simulink model "robotarm_A2_breach"  (R2018b)
settings: Solver=FixedStepAuto  StartTime=0.0  StopTime=tspan(end)  RelTol=1e-3  AbsTol=1e-6
undefined symbols (not defined in the file): options
libraries: neural x132, simulink x2
(part 2 of 6)

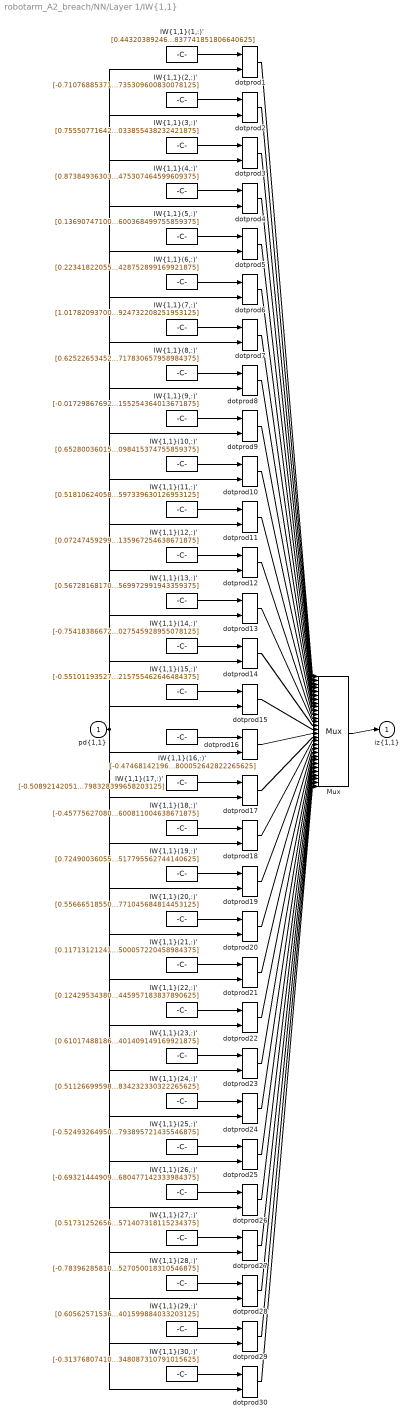
== system robotarm_A2_breach/NN/Layer 1/IW{1,1} ==
  "pd{1,1}" : Inport  PortDimensions=10
      mask Display: e = 0.06;c1 = [120 230 180]/255;c2 = ([120 230 180]+0)/(256+128);c3 = ([120 230 180]+128)/(256+128);patch([0 1 1 0],[0 0 1 1],c1);patch([0 1 1 1-e 1-e 0+e],[0 0 1 1-e 0+e 0+e],c2);patch([0 0 1 1-e 0+e 0+e],[0 1 1 1-e 1-e 0+e],c3);plot([0 1 1 0 0],[0 0 1 1 0]);
  "IW{1,1}(1,:)'" : Constant  Value=[0.44320389246650415682182710952474735677242279052734375;0.51947584556928483312532307536457665264606475830078125;-0.1013749825861565978524225783985457383096218109130859375;-0.465941513924777728217208050409681163728237152099609375;0.67801884953176971837507380769238807260990142822265625;-0.81570216281103657962603392661549150943756103515625;0.80632098302361898678469742662855423986911773681640625;0.01324690942009895851250167453372341697104275226593017578125;-0.64580771410095449969190894989878870546817779541015625;-0.76009607664536960047740876689204014837741851806640625]
      mask Display: e = 0.06;c1 = [120 150 230]/255;c2 = ([120 150 230]+0)/383;c3 = ([120 150 230]+128)/383;patch([0 1 1 0],[0 0 1 1],c1);patch([0 1 1 1-e 1-e 0+e],[0 0 1 1-e 0+e 0+e],c2);patch([0 0 1 1-e 0+e 0+e],[0 1 1 1-e 1-e 0+e],c3);plot([0 1 1 0 0],[0 0 1 1 0]);disp('Weights');
  "IW{1,1}(10,:)'" : Constant  Value=[0.6528003601570897540540272530051879584789276123046875;-0.805642874886827176084125312627293169498443603515625;-0.016554816769301171353045987189034349285066127777099609375;0.76137713758309855105466112945578061044216156005859375;-0.7006051933474084503217227393179200589656829833984375;0.7652873118121277240533117947052232921123504638671875;0.51417600395731877238603146906825713813304901123046875;0.247761309628450943076671819653711281716823577880859375;0.349447996093606771950135225779376924037933349609375;0.8974588918394699188496588249108754098415374755859375]
      mask Display: e = 0.06;c1 = [120 150 230]/255;c2 = ([120 150 230]+0)/383;c3 = ([120 150 230]+128)/383;patch([0 1 1 0],[0 0 1 1],c1);patch([0 1 1 1-e 1-e 0+e],[0 0 1 1-e 0+e 0+e],c2);patch([0 0 1 1-e 0+e 0+e],[0 1 1 1-e 1-e 0+e],c3);plot([0 1 1 0 0],[0 0 1 1 0]);disp('Weights');
  "IW{1,1}(11,:)'" : Constant  Value=[0.51810624058172383143983097397722303867340087890625;0.872191799817235047243002554751001298427581787109375;-0.712884895735269363825636901310645043849945068359375;0.002494892009457406502337395437507439055480062961578369140625;-0.270486052055616099654145045860786922276020050048828125;0.6707615472857841876219708865392021834850311279296875;0.0246310505931925417810735012835721136070787906646728515625;0.77266353199085024971992652353947050869464874267578125;-0.3568298560395135599065952192177064716815948486328125;0.360121164362003032266557056573219597339630126953125]
      mask Display: e = 0.06;c1 = [120 150 230]/255;c2 = ([120 150 230]+0)/383;c3 = ([120 150 230]+128)/383;patch([0 1 1 0],[0 0 1 1],c1);patch([0 1 1 1-e 1-e 0+e],[0 0 1 1-e 0+e 0+e],c2);patch([0 0 1 1-e 0+e 0+e],[0 1 1 1-e 1-e 0+e],c3);plot([0 1 1 0 0],[0 0 1 1 0]);disp('Weights');
  "IW{1,1}(12,:)'" : Constant  Value=[0.07247459299068963189949243997034500353038311004638671875;0.77588832922420791771145331949810497462749481201171875;-0.01498952312966151008410964351469374378211796283721923828125;-0.66950481581926502006041346248821355402469635009765625;-1.0394647414620890035763522973866201937198638916015625;0.41659107015939067508725202060304582118988037109375;-0.56564242470902581505498574188095517456531524658203125;0.772999076426951869933645866694860160350799560546875;-0.15300878050934751950507006768020801246166229248046875;0.46525515641211512285480011996696703135967254638671875]
      mask Display: e = 0.06;c1 = [120 150 230]/255;c2 = ([120 150 230]+0)/383;c3 = ([120 150 230]+128)/383;patch([0 1 1 0],[0 0 1 1],c1);patch([0 1 1 1-e 1-e 0+e],[0 0 1 1-e 0+e 0+e],c2);patch([0 0 1 1-e 0+e 0+e],[0 1 1 1-e 1-e 0+e],c3);plot([0 1 1 0 0],[0 0 1 1 0]);disp('Weights');
  "IW{1,1}(13,:)'" : Constant  Value=[0.56728168170493098454443270384217612445354461669921875;0.277793118270089234300712632830254733562469482421875;-0.5975587782155187266397433631937019526958465576171875;0.06833884407195851828920041270976071245968341827392578125;-0.856917725762365467545578212593682110309600830078125;0.7908637356047483191190394791192375123500823974609375;-0.06487009020830931949053166363228228874504566192626953125;0.2372887359075701863009300041085225529968738555908203125;-0.2256653137890034799273308863121201284229755401611328125;0.8783771195165426259876539916149340569972991943359375]
      mask Display: e = 0.06;c1 = [120 150 230]/255;c2 = ([120 150 230]+0)/383;c3 = ([120 150 230]+128)/383;patch([0 1 1 0],[0 0 1 1],c1);patch([0 1 1 1-e 1-e 0+e],[0 0 1 1-e 0+e 0+e],c2);patch([0 0 1 1-e 0+e 0+e],[0 1 1 1-e 1-e 0+e],c3);plot([0 1 1 0 0],[0 0 1 1 0]);disp('Weights');
  "IW{1,1}(14,:)'" : Constant  Value=[-0.75418386672222437194790245484909974038600921630859375;1.1398123201737184739812391853774897754192352294921875;-0.58445642008161347025207987826433964073657989501953125;0.164696959702814005321869217368657700717449188232421875;-0.73703910480042511554898965187021531164646148681640625;0.471437080031712529848419990230468101799488067626953125;0.59769416587250834282940559205599129199981689453125;0.018010030288912466656103816831091535277664661407470703125;-0.377438339776456188712216999192605726420879364013671875;0.111431025352921431181840716817532666027545928955078125]
      mask Display: e = 0.06;c1 = [120 150 230]/255;c2 = ([120 150 230]+0)/383;c3 = ([120 150 230]+128)/383;patch([0 1 1 0],[0 0 1 1],c1);patch([0 1 1 1-e 1-e 0+e],[0 0 1 1-e 0+e 0+e],c2);patch([0 0 1 1-e 0+e 0+e],[0 1 1 1-e 1-e 0+e],c3);plot([0 1 1 0 0],[0 0 1 1 0]);disp('Weights');
  "IW{1,1}(15,:)'" : Constant  Value=[-0.55101193527417435813475776740233413875102996826171875;0.0671325813779753699517272025332204066216945648193359375;-0.60519616319179825314478193831746466457843780517578125;0.58769100257684769861299400872667320072650909423828125;-0.08797219520669753711761273962110863067209720611572265625;-0.5524094229546279155584898035158403217792510986328125;-0.7448941576311882695193844483583234250545501708984375;0.81814789464563464349566856981255114078521728515625;0.5804459365944396598280263788183219730854034423828125;0.8181125456554683150756090981303714215755462646484375]
      mask Display: e = 0.06;c1 = [120 150 230]/255;c2 = ([120 150 230]+0)/383;c3 = ([120 150 230]+128)/383;patch([0 1 1 0],[0 0 1 1],c1);patch([0 1 1 1-e 1-e 0+e],[0 0 1 1-e 0+e 0+e],c2);patch([0 0 1 1-e 0+e 0+e],[0 1 1 1-e 1-e 0+e],c3);plot([0 1 1 0 0],[0 0 1 1 0]);disp('Weights');
  "IW{1,1}(16,:)'" : Constant  Value=[-0.4746814219666923850837747522746212780475616455078125;0.94193468075639363856765839955187402665615081787109375;-0.81513375864305803730758270830847322940826416015625;-0.5388084969969246795784556525177322328090667724609375;-0.1592610235542184782264740761092980392277240753173828125;-0.0600385525680668108439164143419475294649600982666015625;-0.329608468077444427546396354955504648387432098388671875;0.584753683074171082267866950132884085178375244140625;-0.51700864122426237745600019479752518236637115478515625;-0.78562921103160709979107423350797034800052642822265625]
      mask Display: e = 0.06;c1 = [120 150 230]/255;c2 = ([120 150 230]+0)/383;c3 = ([120 150 230]+128)/383;patch([0 1 1 0],[0 0 1 1],c1);patch([0 1 1 1-e 1-e 0+e],[0 0 1 1-e 0+e 0+e],c2);patch([0 0 1 1-e 0+e 0+e],[0 1 1 1-e 1-e 0+e],c3);plot([0 1 1 0 0],[0 0 1 1 0]);disp('Weights');
  "IW{1,1}(17,:)'" : Constant  Value=[-0.50892142051125277557588333365856669843196868896484375;-0.69555083700712694305678951423033140599727630615234375;0.60851594624274041311906557893962599337100982666015625;-1.0252220281550294966876890612184070050716400146484375;-0.2168840042489936503766756459299358539283275604248046875;0.6757041508143555308407712800544686615467071533203125;0.479959671170491375402633593694190494716167449951171875;-0.792943564626870767142463591881096363067626953125;0.1627362166961741907211802526944666169583797454833984375;0.0198821736009527801070095875957122188992798328399658203125]
      mask Display: e = 0.06;c1 = [120 150 230]/255;c2 = ([120 150 230]+0)/383;c3 = ([120 150 230]+128)/383;patch([0 1 1 0],[0 0 1 1],c1);patch([0 1 1 1-e 1-e 0+e],[0 0 1 1-e 0+e 0+e],c2);patch([0 0 1 1-e 0+e 0+e],[0 1 1 1-e 1-e 0+e],c3);plot([0 1 1 0 0],[0 0 1 1 0]);disp('Weights');
  "IW{1,1}(18,:)'" : Constant  Value=[-0.4577562708069302654934062957181595265865325927734375;1.2676395565921485530935797214624471962451934814453125;0.364524994376268285378728251089341938495635986328125;0.316539673426614542872670199358253739774227142333984375;0.1632538241122458988474619445696589536964893341064453125;0.49761099855925594592775951241492293775081634521484375;-0.748043169166599408725915054674260318279266357421875;0.275886447527427247639053575767320580780506134033203125;-0.27855783778322640298341639208956621587276458740234375;0.46158990380921494089960788187454454600811004638671875]
      mask Display: e = 0.06;c1 = [120 150 230]/255;c2 = ([120 150 230]+0)/383;c3 = ([120 150 230]+128)/383;patch([0 1 1 0],[0 0 1 1],c1);patch([0 1 1 1-e 1-e 0+e],[0 0 1 1-e 0+e 0+e],c2);patch([0 0 1 1-e 0+e 0+e],[0 1 1 1-e 1-e 0+e],c3);plot([0 1 1 0 0],[0 0 1 1 0]);disp('Weights');
  "IW{1,1}(19,:)'" : Constant  Value=[0.724900360550514211155359589611180126667022705078125;-0.74523780018478535946968577263760380446910858154296875;-0.47796223974658491595590703582274727523326873779296875;0.322867547667288146140407434359076432883739471435546875;0.50749193517804369601975622572354041039943695068359375;0.79033776973074820748621505117625929415225982666015625;-0.4530942934193140647636255380348302423954010009765625;-0.499085576358067106728100270629511214792728424072265625;0.139279961878759628302049122794414870440959930419921875;0.2482889911062852450474025545190670527517795562744140625]
      mask Display: e = 0.06;c1 = [120 150 230]/255;c2 = ([120 150 230]+0)/383;c3 = ([120 150 230]+128)/383;patch([0 1 1 0],[0 0 1 1],c1);patch([0 1 1 1-e 1-e 0+e],[0 0 1 1-e 0+e 0+e],c2);patch([0 0 1 1-e 0+e 0+e],[0 1 1 1-e 1-e 0+e],c3);plot([0 1 1 0 0],[0 0 1 1 0]);disp('Weights');
  "IW{1,1}(2,:)'" : Constant  Value=[-0.71076885371394282753243487604777328670024871826171875;-0.7199239242746739986245074760518036782741546630859375;0.60890423360056422641406470575020648539066314697265625;-0.8359265181922317378138131971354596316814422607421875;-0.01236466893263855719442556591047832625918090343475341796875;-0.086936016752006739505276300405967049300670623779296875;-0.83008311124606082298527098828344605863094329833984375;-0.708547490288692127791136954328976571559906005859375;-0.372731541127455046069627542237867601215839385986328125;0.6533615363197065040168354244087822735309600830078125]
      mask Display: e = 0.06;c1 = [120 150 230]/255;c2 = ([120 150 230]+0)/383;c3 = ([120 150 230]+128)/383;patch([0 1 1 0],[0 0 1 1],c1);patch([0 1 1 1-e 1-e 0+e],[0 0 1 1-e 0+e 0+e],c2);patch([0 0 1 1-e 0+e 0+e],[0 1 1 1-e 1-e 0+e],c3);plot([0 1 1 0 0],[0 0 1 1 0]);disp('Weights');
  "IW{1,1}(20,:)'" : Constant  Value=[0.5566651855048128094693993261898867785930633544921875;-0.44166086307228591412155083162360824644565582275390625;0.047687377290480836844466239199391566216945648193359375;-0.58969305305443875386828267437522299587726593017578125;-0.27878213042887522998825033937464468181133270263671875;0.95487524421580893818628510416601784527301788330078125;-0.3976653837847201611310765656526200473308563232421875;0.2471805959416451814458781655048369430005550384521484375;-0.18325039106971008351365526323206722736358642578125;0.5749228586424852682768005252000875771045684814453125]
      mask Display: e = 0.06;c1 = [120 150 230]/255;c2 = ([120 150 230]+0)/383;c3 = ([120 150 230]+128)/383;patch([0 1 1 0],[0 0 1 1],c1);patch([0 1 1 1-e 1-e 0+e],[0 0 1 1-e 0+e 0+e],c2);patch([0 0 1 1-e 0+e 0+e],[0 1 1 1-e 1-e 0+e],c3);plot([0 1 1 0 0],[0 0 1 1 0]);disp('Weights');
  "IW{1,1}(21,:)'" : Constant  Value=[0.11713121241022854401858666051339241676032543182373046875;-0.161379468950165361196269486754317767918109893798828125;-0.7571548590667889211403007720946334302425384521484375;-0.5838206531095664342245754596660844981670379638671875;-0.239675887371985696372433949363767169415950775146484375;-0.4271977908733119999595828630845062434673309326171875;-0.5864204481509058819455049160751514136791229248046875;0.832557507211043823502905070199631154537200927734375;-0.43356891709465716910898436253773979842662811279296875;-0.6054667698450602042470336527912877500057220458984375]
      mask Display: e = 0.06;c1 = [120 150 230]/255;c2 = ([120 150 230]+0)/383;c3 = ([120 150 230]+128)/383;patch([0 1 1 0],[0 0 1 1],c1);patch([0 1 1 1-e 1-e 0+e],[0 0 1 1-e 0+e 0+e],c2);patch([0 0 1 1-e 0+e 0+e],[0 1 1 1-e 1-e 0+e],c3);plot([0 1 1 0 0],[0 0 1 1 0]);disp('Weights');
  "IW{1,1}(22,:)'" : Constant  Value=[0.1242953438074253791345569197801523841917514801025390625;0.8801330808879919143095094113959930837154388427734375;-0.63780439820036083364840351350721903145313262939453125;-0.33948603439440550033623367198742926120758056640625;0.4331515967100065811479225885705091059207916259765625;0.78263969117551901444329587320680730044841766357421875;0.361190678789260755099377320220810361206531524658203125;-0.89372467515034514917715569026768207550048828125;-0.6160858098907056046300567686557769775390625;-0.1207696284431253597180244696573936380445957183837890625]
      mask Display: e = 0.06;c1 = [120 150 230]/255;c2 = ([120 150 230]+0)/383;c3 = ([120 150 230]+128)/383;patch([0 1 1 0],[0 0 1 1],c1);patch([0 1 1 1-e 1-e 0+e],[0 0 1 1-e 0+e 0+e],c2);patch([0 0 1 1-e 0+e 0+e],[0 1 1 1-e 1-e 0+e],c3);plot([0 1 1 0 0],[0 0 1 1 0]);disp('Weights');
  "IW{1,1}(23,:)'" : Constant  Value=[0.61017488186100854452575958930538035929203033447265625;0.1706451267918588643457411535564460791647434234619140625;-0.458039832655668111005553555514779873192310333251953125;-0.65247583865402258851418082485906779766082763671875;0.5436317432158996876268020059796981513500213623046875;-0.57938981805185096884969198072212748229503631591796875;0.6548718804419044747788802851573564112186431884765625;0.1616631179037730514647108748249593190848827362060546875;-0.727430760154359479230379292857833206653594970703125;0.541767729955985100076532035018317401409149169921875]
      mask Display: e = 0.06;c1 = [120 150 230]/255;c2 = ([120 150 230]+0)/383;c3 = ([120 150 230]+128)/383;patch([0 1 1 0],[0 0 1 1],c1);patch([0 1 1 1-e 1-e 0+e],[0 0 1 1-e 0+e 0+e],c2);patch([0 0 1 1-e 0+e 0+e],[0 1 1 1-e 1-e 0+e],c3);plot([0 1 1 0 0],[0 0 1 1 0]);disp('Weights');
  "IW{1,1}(24,:)'" : Constant  Value=[0.51126699598210845199020013751578517258167266845703125;0.2474125636719124166074124104852671734988689422607421875;0.7825633408629191212213527251151390373706817626953125;0.401031003354632542556856833471101708710193634033203125;0.40237460000039659835380234653712250292301177978515625;0.428379990475945049421824251112411729991436004638671875;0.78279557710397240644084604355157352983951568603515625;-0.79848599732739600209896480009774677455425262451171875;-0.164755224531509092411596384408767335116863250732421875;-0.54600511891358627369896794334636069834232330322265625]
      mask Display: e = 0.06;c1 = [120 150 230]/255;c2 = ([120 150 230]+0)/383;c3 = ([120 150 230]+128)/383;patch([0 1 1 0],[0 0 1 1],c1);patch([0 1 1 1-e 1-e 0+e],[0 0 1 1-e 0+e 0+e],c2);patch([0 0 1 1-e 0+e 0+e],[0 1 1 1-e 1-e 0+e],c3);plot([0 1 1 0 0],[0 0 1 1 0]);disp('Weights');
  "IW{1,1}(25,:)'" : Constant  Value=[-0.524932649501538950431722696521319448947906494140625;-0.648777122723714239072023701737634837627410888671875;0.0307647862348335542070909554013269371353089809417724609375;0.6454191306393770588556435541249811649322509765625;-0.5017327542510103821626898934482596814632415771484375;0.99523431649100546625419383417465724050998687744140625;-0.75566215465000008411067256020032800734043121337890625;-0.070746109627535691544153451104648411273956298828125;-0.01490998250299602201351945041096769273281097412109375;-0.52465858272687693197866565242293290793895721435546875]
      mask Display: e = 0.06;c1 = [120 150 230]/255;c2 = ([120 150 230]+0)/383;c3 = ([120 150 230]+128)/383;patch([0 1 1 0],[0 0 1 1],c1);patch([0 1 1 1-e 1-e 0+e],[0 0 1 1-e 0+e 0+e],c2);patch([0 0 1 1-e 0+e 0+e],[0 1 1 1-e 1-e 0+e],c3);plot([0 1 1 0 0],[0 0 1 1 0]);disp('Weights');
  "IW{1,1}(26,:)'" : Constant  Value=[-0.69321444909777196752287409253767691552639007568359375;0.310984724690046399064868865025346167385578155517578125;-0.69058813895924486825350641083787195384502410888671875;-0.70125747804459270806631820960319600999355316162109375;0.27626987322017981796307140029966831207275390625;-0.284795830435694174997962591078248806297779083251953125;0.038821887770207667844868382189815747551620006561279296875;-0.71972748404353625861773480210104025900363922119140625;-0.39656616262824850860368997018667869269847869873046875;-0.73129209094150071646112110101967118680477142333984375]
      mask Display: e = 0.06;c1 = [120 150 230]/255;c2 = ([120 150 230]+0)/383;c3 = ([120 150 230]+128)/383;patch([0 1 1 0],[0 0 1 1],c1);patch([0 1 1 1-e 1-e 0+e],[0 0 1 1-e 0+e 0+e],c2);patch([0 0 1 1-e 0+e 0+e],[0 1 1 1-e 1-e 0+e],c3);plot([0 1 1 0 0],[0 0 1 1 0]);disp('Weights');
  "IW{1,1}(27,:)'" : Constant  Value=[0.5173125265682563256319781430647708475589752197265625;-0.049397491354776119909519849215939757414162158966064453125;-0.81740761486488278109163729823194444179534912109375;-0.08412318439210035581066193799415486864745616912841796875;0.1553109267276908955768277564857271499931812286376953125;0.17722402391180158698347213430679403245449066162109375;-0.90548653814202573197889023504103533923625946044921875;0.41262963643356564968911470714374445378780364990234375;1.087835541343836087690988279064185917377471923828125;0.56545162151599848154859273563488386571407318115234375]
      mask Display: e = 0.06;c1 = [120 150 230]/255;c2 = ([120 150 230]+0)/383;c3 = ([120 150 230]+128)/383;patch([0 1 1 0],[0 0 1 1],c1);patch([0 1 1 1-e 1-e 0+e],[0 0 1 1-e 0+e 0+e],c2);patch([0 0 1 1-e 0+e 0+e],[0 1 1 1-e 1-e 0+e],c3);plot([0 1 1 0 0],[0 0 1 1 0]);disp('Weights');
  "IW{1,1}(28,:)'" : Constant  Value=[-0.78396285810341759248132120774243958294391632080078125;-0.00910046633940105216542537647228527930565178394317626953125;-0.66004759121113687481141596435918472707271575927734375;-0.78043938724562778030957588271121494472026824951171875;-0.2491602188595275768623338308316306211054325103759765625;0.68534921788892899652267942656180821359157562255859375;-0.0069191367098792866396905765213887207210063934326171875;-0.84621331274527544774599618904176168143749237060546875;0.5373132351323077759985835655243135988712310791015625;0.62345550018999773556060972623527050018310546875]
      mask Display: e = 0.06;c1 = [120 150 230]/255;c2 = ([120 150 230]+0)/383;c3 = ([120 150 230]+128)/383;patch([0 1 1 0],[0 0 1 1],c1);patch([0 1 1 1-e 1-e 0+e],[0 0 1 1-e 0+e 0+e],c2);patch([0 0 1 1-e 0+e 0+e],[0 1 1 1-e 1-e 0+e],c3);plot([0 1 1 0 0],[0 0 1 1 0]);disp('Weights');
  "IW{1,1}(29,:)'" : Constant  Value=[0.60562571536392340032506353963981382548809051513671875;-0.532825242205438254217142457491718232631683349609375;0.82195499843903763181884869482018984854221343994140625;-0.1673989818227205883527375362973543815314769744873046875;0.68771892273064205713950514109455980360507965087890625;-0.09491219601184143483951771713691414333879947662353515625;-0.48907899718634617602930347857181914150714874267578125;0.34930477962741812714142497497959993779659271240234375;-0.497850007887704337772305507314740680158138275146484375;1.07647261589812348603345526498742401599884033203125]
      mask Display: e = 0.06;c1 = [120 150 230]/255;c2 = ([120 150 230]+0)/383;c3 = ([120 150 230]+128)/383;patch([0 1 1 0],[0 0 1 1],c1);patch([0 1 1 1-e 1-e 0+e],[0 0 1 1-e 0+e 0+e],c2);patch([0 0 1 1-e 0+e 0+e],[0 1 1 1-e 1-e 0+e],c3);plot([0 1 1 0 0],[0 0 1 1 0]);disp('Weights');
  "IW{1,1}(3,:)'" : Constant  Value=[0.75550771642954728246621698417584411799907684326171875;0.4651970624553471989059971747337840497493743896484375;0.316389969701839135485244014489580877125263214111328125;0.95234081392340019789344296441413462162017822265625;-0.54512424096975220511041015925002284348011016845703125;-0.1199486488292370311992129927602945826947689056396484375;-0.489955622693164671854759717462002299726009368896484375;-0.25132352667878044005789206494227983057498931884765625;0.1268370320189154132339837133258697576820850372314453125;-0.744428647658245790097453209455125033855438232421875]
      mask Display: e = 0.06;c1 = [120 150 230]/255;c2 = ([120 150 230]+0)/383;c3 = ([120 150 230]+128)/383;patch([0 1 1 0],[0 0 1 1],c1);patch([0 1 1 1-e 1-e 0+e],[0 0 1 1-e 0+e 0+e],c2);patch([0 0 1 1-e 0+e 0+e],[0 1 1 1-e 1-e 0+e],c3);plot([0 1 1 0 0],[0 0 1 1 0]);disp('Weights');
  "IW{1,1}(30,:)'" : Constant  Value=[-0.313768074103874361480137622493202798068523406982421875;-0.617033842266395904374576275586150586605072021484375;0.410502019716686927797155703956377692520618438720703125;0.81012929193932325944160766084678471088409423828125;-0.043151646587668519849945170108185266144573688507080078125;0.0210179663767442910515814702421266702003777027130126953125;-0.424715750473314390678325480621424503624439239501953125;0.88620338133446885375832380304927937686443328857421875;-0.7949468812020141772478609709651209414005279541015625;0.93967254890675688816514821155578829348087310791015625]
      mask Display: e = 0.06;c1 = [120 150 230]/255;c2 = ([120 150 230]+0)/383;c3 = ([120 150 230]+128)/383;patch([0 1 1 0],[0 0 1 1],c1);patch([0 1 1 1-e 1-e 0+e],[0 0 1 1-e 0+e 0+e],c2);patch([0 0 1 1-e 0+e 0+e],[0 1 1 1-e 1-e 0+e],c3);plot([0 1 1 0 0],[0 0 1 1 0]);disp('Weights');
  "IW{1,1}(4,:)'" : Constant  Value=[0.87384936303111848676650197376147843897342681884765625;-0.2287493200660979109084536275986465625464916229248046875;-0.241602336087604452341537353277090005576610565185546875;-0.1587639918776705127978488008011481724679470062255859375;-0.95146944816727463400951592120691202580928802490234375;-0.60279055737714148932582247653044760227203369140625;0.6273114429944215419965303226490505039691925048828125;0.57828806947814526129292289624572731554508209228515625;0.34936344574905942028664185272646136581897735595703125;-0.023795202179214401672080470007131225429475307464599609375]
      mask Display: e = 0.06;c1 = [120 150 230]/255;c2 = ([120 150 230]+0)/383;c3 = ([120 150 230]+128)/383;patch([0 1 1 0],[0 0 1 1],c1);patch([0 1 1 1-e 1-e 0+e],[0 0 1 1-e 0+e 0+e],c2);patch([0 0 1 1-e 0+e 0+e],[0 1 1 1-e 1-e 0+e],c3);plot([0 1 1 0 0],[0 0 1 1 0]);disp('Weights');
  "IW{1,1}(5,:)'" : Constant  Value=[0.1369074710004203609958750575970043428242206573486328125;-0.1139511764867985055271759620154625736176967620849609375;1.0525915567382597703982582970638759434223175048828125;-0.298822917521910202953705493200686760246753692626953125;-0.97249453951210573787733437711722217500209808349609375;0.79674479353023475169948142138309776782989501953125;-0.1330203219585482099507345310485106892883777618408203125;-0.6436253507153135711149616327020339667797088623046875;0.266075168516050009070994519788655452430248260498046875;0.02548060304491460426046245402176282368600368499755859375]
      mask Display: e = 0.06;c1 = [120 150 230]/255;c2 = ([120 150 230]+0)/383;c3 = ([120 150 230]+128)/383;patch([0 1 1 0],[0 0 1 1],c1);patch([0 1 1 1-e 1-e 0+e],[0 0 1 1-e 0+e 0+e],c2);patch([0 0 1 1-e 0+e 0+e],[0 1 1 1-e 1-e 0+e],c3);plot([0 1 1 0 0],[0 0 1 1 0]);disp('Weights');
  "IW{1,1}(6,:)'" : Constant  Value=[0.2234182205573691515354539660620503127574920654296875;-0.86690746220813375000346923116012476384639739990234375;0.94444867744370719631064048371626995503902435302734375;1.074067905807680300966922004590742290019989013671875;0.2481737568000013383073820705249090678989887237548828125;-0.261006977650531102330688781876233406364917755126953125;-0.380288866215888032851211164597771130502223968505859375;-0.25353732613580215460302724750363267958164215087890625;0.638937860708570948276019407785497605800628662109375;0.1333282944150208926270551046400214545428752899169921875]
      mask Display: e = 0.06;c1 = [120 150 230]/255;c2 = ([120 150 230]+0)/383;c3 = ([120 150 230]+128)/383;patch([0 1 1 0],[0 0 1 1],c1);patch([0 1 1 1-e 1-e 0+e],[0 0 1 1-e 0+e 0+e],c2);patch([0 0 1 1-e 0+e 0+e],[0 1 1 1-e 1-e 0+e],c3);plot([0 1 1 0 0],[0 0 1 1 0]);disp('Weights');
  "IW{1,1}(7,:)'" : Constant  Value=[1.017820937001784553643801700673066079616546630859375;0.40855130381393911509491090328083373606204986572265625;0.397315672322906709990064655357855372130870819091796875;0.01521358336158879810684485534011400886811316013336181640625;0.07800441716808721726028608145497855730354785919189453125;-0.1554513220874771117774315598580869846045970916748046875;0.5621451195729696426184318625018931925296783447265625;0.7946680824603458148658319259993731975555419921875;0.53650469033950487496298364931135438382625579833984375;-0.51599999329390844327036802496877498924732208251953125]
      mask Display: e = 0.06;c1 = [120 150 230]/255;c2 = ([120 150 230]+0)/383;c3 = ([120 150 230]+128)/383;patch([0 1 1 0],[0 0 1 1],c1);patch([0 1 1 1-e 1-e 0+e],[0 0 1 1-e 0+e 0+e],c2);patch([0 0 1 1-e 0+e 0+e],[0 1 1 1-e 1-e 0+e],c3);plot([0 1 1 0 0],[0 0 1 1 0]);disp('Weights');
  "IW{1,1}(8,:)'" : Constant  Value=[0.62522653452871035373306085602962411940097808837890625;-0.62499448228666754090454560355283319950103759765625;-0.6579888802018782900660198720288462936878204345703125;0.417744195494852477157365910898079164326190948486328125;-0.717550952346133197323752028751187026500701904296875;0.4652313896980599938757450217963196337223052978515625;-0.7028735615850560947137637413106858730316162109375;0.269824973790782574045721275979303754866123199462890625;-0.80052495489638175740765291266143321990966796875;0.2878933218308306063448753775446675717830657958984375]
      mask Display: e = 0.06;c1 = [120 150 230]/255;c2 = ([120 150 230]+0)/383;c3 = ([120 150 230]+128)/383;patch([0 1 1 0],[0 0 1 1],c1);patch([0 1 1 1-e 1-e 0+e],[0 0 1 1-e 0+e 0+e],c2);patch([0 0 1 1-e 0+e 0+e],[0 1 1 1-e 1-e 0+e],c3);plot([0 1 1 0 0],[0 0 1 1 0]);disp('Weights');
  "IW{1,1}(9,:)'" : Constant  Value=[-0.0172986769296754640257152146887165145017206668853759765625;-0.5329186140946335914492237861850298941135406494140625;0.61939908834851842289737078317557461559772491455078125;-0.329992727773426308690574160209507681429386138916015625;-1.0193204469705381409738720321911387145519256591796875;0.81164190044688344638501575900590978562831878662109375;-0.11180129901829237437649311459608725272119045257568359375;0.36683924979239213026716015519923530519008636474609375;-0.6534477435602068506881323628476820886135101318359375;-0.05659662109145240094232320871014962904155254364013671875]
      mask Display: e = 0.06;c1 = [120 150 230]/255;c2 = ([120 150 230]+0)/383;c3 = ([120 150 230]+128)/383;patch([0 1 1 0],[0 0 1 1],c1);patch([0 1 1 1-e 1-e 0+e],[0 0 1 1-e 0+e 0+e],c2);patch([0 0 1 1-e 0+e 0+e],[0 1 1 1-e 1-e 0+e],c3);plot([0 1 1 0 0],[0 0 1 1 0]);disp('Weights');
  Mux : Mux  Inputs=30
      mask Display: e = 0.06;c1 = [120 150 230]/255;c2 = ([120 150 230]+0)/383;c3 = ([120 150 230]+128)/383;patch([0 1 1 0],[0 0 1 1],c1);patch([0 1 1 1-e 1-e 0+e],[0 0 1 1-e 0+e 0+e],c2);patch([0 0 1 1-e 0+e 0+e],[0 1 1 1-e 1-e 0+e],c3);plot([0 1 1 0 0],[0 0 1 1 0]);disp('Mux');
  dotprod{1..30} (30 alike) : neural/Weight Functions/dotprod
  "iz{1,1}" : Outport
      mask Display: e = 0.06;c1 = [120 230 180]/255;c2 = ([120 230 180]+0)/(256+128);c3 = ([120 230 180]+128)/(256+128);patch([0 1 1 0],[0 0 1 1],c1);patch([0 1 1 1-e 1-e 0+e],[0 0 1 1-e 0+e 0+e],c2);patch([0 0 1 1-e 0+e 0+e],[0 1 1 1-e 1-e 0+e],c3);plot([0 1 1 0 0],[0 0 1 1 0]);
  wires:
  "IW{1,1}(1,:)'"/1 -> dotprod1/1
  "pd{1,1}"/1 -> dotprod1/2, dotprod2/2, dotprod3/2, dotprod4/2, dotprod5/2, dotprod6/2, dotprod7/2, dotprod8/2, dotprod9/2, dotprod10/2, dotprod11/2, dotprod12/2, dotprod13/2, dotprod14/2, dotprod15/2, dotprod16/2, dotprod17/2, dotprod18/2, dotprod19/2, dotprod20/2, dotprod21/2, dotprod22/2, dotprod23/2, dotprod24/2, dotprod25/2, dotprod26/2, dotprod27/2, dotprod28/2, dotprod29/2, dotprod30/2
  dotprod1/1 -> Mux/1
  "IW{1,1}(2,:)'"/1 -> dotprod2/1
  dotprod2/1 -> Mux/2
  "IW{1,1}(3,:)'"/1 -> dotprod3/1
  dotprod3/1 -> Mux/3
  "IW{1,1}(4,:)'"/1 -> dotprod4/1
  dotprod4/1 -> Mux/4
  "IW{1,1}(5,:)'"/1 -> dotprod5/1
  dotprod5/1 -> Mux/5
  "IW{1,1}(6,:)'"/1 -> dotprod6/1
  dotprod6/1 -> Mux/6
  "IW{1,1}(7,:)'"/1 -> dotprod7/1
  dotprod7/1 -> Mux/7
  "IW{1,1}(8,:)'"/1 -> dotprod8/1
  dotprod8/1 -> Mux/8
  "IW{1,1}(9,:)'"/1 -> dotprod9/1
  dotprod9/1 -> Mux/9
  "IW{1,1}(10,:)'"/1 -> dotprod10/1
  dotprod10/1 -> Mux/10
  "IW{1,1}(11,:)'"/1 -> dotprod11/1
  dotprod11/1 -> Mux/11
  "IW{1,1}(12,:)'"/1 -> dotprod12/1
  dotprod12/1 -> Mux/12
  "IW{1,1}(13,:)'"/1 -> dotprod13/1
  dotprod13/1 -> Mux/13
  "IW{1,1}(14,:)'"/1 -> dotprod14/1
  dotprod14/1 -> Mux/14
  "IW{1,1}(15,:)'"/1 -> dotprod15/1
  dotprod15/1 -> Mux/15
  "IW{1,1}(16,:)'"/1 -> dotprod16/1
  dotprod16/1 -> Mux/16
  "IW{1,1}(17,:)'"/1 -> dotprod17/1
  dotprod17/1 -> Mux/17
  "IW{1,1}(18,:)'"/1 -> dotprod18/1
  dotprod18/1 -> Mux/18
  "IW{1,1}(19,:)'"/1 -> dotprod19/1
  dotprod19/1 -> Mux/19
  "IW{1,1}(20,:)'"/1 -> dotprod20/1
  dotprod20/1 -> Mux/20
  "IW{1,1}(21,:)'"/1 -> dotprod21/1
  dotprod21/1 -> Mux/21
  "IW{1,1}(22,:)'"/1 -> dotprod22/1
  dotprod22/1 -> Mux/22
  "IW{1,1}(23,:)'"/1 -> dotprod23/1
  dotprod23/1 -> Mux/23
  "IW{1,1}(24,:)'"/1 -> dotprod24/1
  dotprod24/1 -> Mux/24
  "IW{1,1}(25,:)'"/1 -> dotprod25/1
  dotprod25/1 -> Mux/25
  "IW{1,1}(26,:)'"/1 -> dotprod26/1
  dotprod26/1 -> Mux/26
  "IW{1,1}(27,:)'"/1 -> dotprod27/1
  dotprod27/1 -> Mux/27
  "IW{1,1}(28,:)'"/1 -> dotprod28/1
  dotprod28/1 -> Mux/28
  "IW{1,1}(29,:)'"/1 -> dotprod29/1
  dotprod29/1 -> Mux/29
  "IW{1,1}(30,:)'"/1 -> dotprod30/1
  dotprod30/1 -> Mux/30
  Mux/1 -> "iz{1,1}"/1

== system robotarm_A2_breach/NN/Layer 2/Delays 1 ==
  "p{2}" : Inport  PortDimensions=30
      mask Display: e = 0.06;c1 = [120 230 180]/255;c2 = ([120 230 180]+0)/(256+128);c3 = ([120 230 180]+128)/(256+128);patch([0 1 1 0],[0 0 1 1],c1);patch([0 1 1 1-e 1-e 0+e],[0 0 1 1-e 0+e 0+e],c2);patch([0 0 1 1-e 0+e 0+e],[0 1 1 1-e 1-e 0+e],c3);plot([0 1 1 0 0],[0 0 1 1 0]);
  mux : Mux  Inputs=1
      mask Display: e = 0.06;c1 = [120 150 230]/255;c2 = ([120 150 230]+0)/383;c3 = ([120 150 230]+128)/383;patch([0 1 1 0],[0 0 1 1],c1);patch([0 1 1 1-e 1-e 0+e],[0 0 1 1-e 0+e 0+e],c2);patch([0 0 1 1-e 0+e 0+e],[0 1 1 1-e 1-e 0+e],c3);plot([0 1 1 0 0],[0 0 1 1 0]);disp('Mux')
  "pd{2,1}" : Outport
      mask Display: e = 0.06;c1 = [120 230 180]/255;c2 = ([120 230 180]+0)/(256+128);c3 = ([120 230 180]+128)/(256+128);patch([0 1 1 0],[0 0 1 1],c1);patch([0 1 1 1-e 1-e 0+e],[0 0 1 1-e 0+e 0+e],c2);patch([0 0 1 1-e 0+e 0+e],[0 1 1 1-e 1-e 0+e],c3);plot([0 1 1 0 0],[0 0 1 1 0]);
  wires:
  "p{2}"/1 -> mux/1
  mux/1 -> "pd{2,1}"/1
